simulink model "eVTOL_System"  (R2024b)
settings: Solver=FixedStepAuto  StartTime=0.0  StopTime=inf  RelTol=1e-3
undefined symbols (not defined in the file): airspeed, Battery, BCE12, BCE_Set_init, BMS_Controller_State, C, Cell10_P, Cell11_P, Cell12_P, Cell13_P, Cell14_P, Cell15_P, Cell16_P, Cell17_P, Cell18_P, Cell19_P, Cell1_N, Cell1_P, Cell20_P, Cell21_P, Cell22_P, Cell23_P, Cell24_P, Cell2_P, Cell3_P, Cell4_P, Cell5_P, Cell6_P, Cell7_P, Cell8_P, Cell9_P, Charging_State, CityMission, control, controlParams, ControlSampleTime, CriticalTiltAngle, currentFactor, CV_Gain, ddx, ddy, ddz, Device_01, Device_02, DiscIntNeverNeededParam, dx, dy, dz, Earth, env, F, F28379D_ADC_MaxCount, F28379D_ADC_Vmax, FixedWingMission, flightState, Foc_Ki_IxTcpu, Foc_Ki_S, Foc_Kp_I, Foc_Kp_S, fractalcoef ... (+68)
libraries: fl_lib x1115, nesl_utility x617, slrealtimeethercatlib x217, simulink x130, canmsglib x101, speedgoatlib_IO611_obsolete x91, slpidlib x49, mcbcontrolslib x44, slrealtimeutilitieslib x35, speedgoatlib_hdlCoder_IO3xx x31, dspstat3 x24, mcbpositiondecoderlib x12
(part 19 of 31)

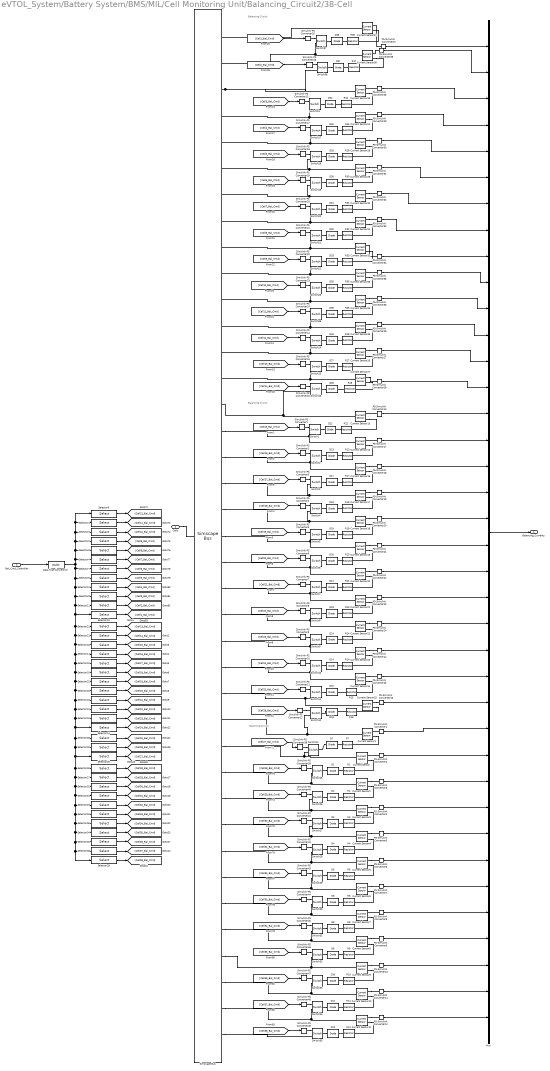
== system eVTOL_System/Battery System/BMS/MIL/Cell Monitoring Unit/Balancing_Circuit2/38-Cell ==
  note: Balancing Circuit
  note: Balancing Circuit
  note: Balancing Circuit
  Bal_Cmd_Controller : Inport
  Current Sensor{,1..37} (38 alike) : fl_lib/Electrical/Electrical Sensors/Current Sensor
  D{1..38} (38 alike) : fl_lib/Electrical/Electrical Elements/Diode  Vf=0.6 V  Ron=0.3 Ohm  Goff=1e-8 1/Ohm  i_specify=off  i_priority=High  i=0 A  i_nominal_specify=off  i_nominal_value=1  i_nominal_unit=A  v_specify=off  v_priority=None  v=0 V  v_nominal_specify=off  v_nominal_value=1  v_nominal_unit=V
      settings: LibrarySourceBlock=BatteryPack_lib/CellMonitoringUnit/D1  LogSimulationData=on
  Data Type Conversion : DataTypeConversion  OutDataTypeStr=double  SaturateOnIntegerOverflow=off  RndMeth=Floor
  Mux : Mux  Inputs=38
  PS-Simulink Converter{1..38} (38 alike) : nesl_utility/PS-Simulink Converter  PhysicalDomain=network_engine_domain  SubClassName=ps_output  LeftPortType=input  RightPortType=output  PseudoPeriodic=off  Frequencies=[]  VectorFormat=inherit  Unit=inherit  AffineConversion=off
  R{1..38} (38 alike) : fl_lib/Electrical/Electrical Elements/Resistor  R=Battery.R_bleed Ohm  i_specify=off  i_priority=None  i=0 A  i_nominal_specify=off  i_nominal_value=1  i_nominal_unit=A  v_specify=off  v_priority=None  v=0 V  v_nominal_specify=off  v_nominal_value=1  v_nominal_unit=V
      settings: LibrarySourceBlock=BatteryPack_lib/CellMonitoringUnit/R1  LogSimulationData=on
  Selector1 : Selector  IndexOptions=Index vector (dialog)  Indices=73  OutputSizes=1
  Selector10 : Selector  IndexOptions=Index vector (dialog)  Indices=63  OutputSizes=1
  Selector11 : Selector  IndexOptions=Index vector (dialog)  Indices=64  OutputSizes=1
  Selector12 : Selector  IndexOptions=Index vector (dialog)  Indices=66  OutputSizes=1
  Selector13 : Selector  IndexOptions=Index vector (dialog)  Indices=76  OutputSizes=1
  Selector14 : Selector  IndexOptions=Index vector (dialog)  Indices=86  OutputSizes=1
  Selector15 : Selector  IndexOptions=Index vector (dialog)  Indices=85  OutputSizes=1
  Selector16 : Selector  IndexOptions=Index vector (dialog)  Indices=83  OutputSizes=1
  Selector17 : Selector  IndexOptions=Index vector (dialog)  Indices=78  OutputSizes=1
  Selector18 : Selector  IndexOptions=Index vector (dialog)  Indices=77  OutputSizes=1
  Selector19 : Selector  IndexOptions=Index vector (dialog)  Indices=80  OutputSizes=1
  Selector2 : Selector  IndexOptions=Index vector (dialog)  Indices=71  OutputSizes=1
  Selector20 : Selector  IndexOptions=Index vector (dialog)  Indices=82  OutputSizes=1
  Selector21 : Selector  IndexOptions=Index vector (dialog)  Indices=75  OutputSizes=1
  Selector22 : Selector  IndexOptions=Index vector (dialog)  Indices=81  OutputSizes=1
  Selector23 : Selector  IndexOptions=Index vector (dialog)  Indices=79  OutputSizes=1
  Selector24 : Selector  IndexOptions=Index vector (dialog)  Indices=84  OutputSizes=1
  Selector25 : Selector  IndexOptions=Index vector (dialog)  Indices=89  OutputSizes=1
  Selector26 : Selector  IndexOptions=Index vector (dialog)  Indices=88  OutputSizes=1
  Selector27 : Selector  IndexOptions=Index vector (dialog)  Indices=91  OutputSizes=1
  Selector29 : Selector  IndexOptions=Index vector (dialog)  Indices=100  OutputSizes=1
  Selector3 : Selector  IndexOptions=Index vector (dialog)  Indices=72  OutputSizes=1
  Selector30 : Selector  IndexOptions=Index vector (dialog)  Indices=98  OutputSizes=1
  Selector31 : Selector  IndexOptions=Index vector (dialog)  Indices=93  OutputSizes=1
  Selector32 : Selector  IndexOptions=Index vector (dialog)  Indices=92  OutputSizes=1
  Selector33 : Selector  IndexOptions=Index vector (dialog)  Indices=95  OutputSizes=1
  Selector34 : Selector  IndexOptions=Index vector (dialog)  Indices=97  OutputSizes=1
  Selector35 : Selector  IndexOptions=Index vector (dialog)  Indices=90  OutputSizes=1
  Selector36 : Selector  IndexOptions=Index vector (dialog)  Indices=96  OutputSizes=1
  Selector37 : Selector  IndexOptions=Index vector (dialog)  Indices=94  OutputSizes=1
  Selector38 : Selector  IndexOptions=Index vector (dialog)  Indices=99  OutputSizes=1
  Selector39 : Selector  IndexOptions=Index vector (dialog)  Indices=87  OutputSizes=1
  Selector4 : Selector  IndexOptions=Index vector (dialog)  Indices=69  OutputSizes=1
  Selector5 : Selector  IndexOptions=Index vector (dialog)  Indices=67  OutputSizes=1
  Selector6 : Selector  IndexOptions=Index vector (dialog)  Indices=74  OutputSizes=1
  Selector7 : Selector  IndexOptions=Index vector (dialog)  Indices=68  OutputSizes=1
  Selector8 : Selector  IndexOptions=Index vector (dialog)  Indices=70  OutputSizes=1
  Selector9 : Selector  IndexOptions=Index vector (dialog)  Indices=65  OutputSizes=1
  Simscape Bus : SimscapeBus  HierarchyStrings=Cell38_P;Cell37_P;Cell36_P;Cell35_P;Cell34_P;Cell33_P;Cell32_P;Cell31_P;Cell30_P;Cell29_P;Cell28_P;Cell27_P;Cell26_P;Cell25_P;Cell24_P;Cell23_P;Cell22_P;Cell21_P;Cell20_P;Cell19_P;Cell18_P;Cell17_P;Cell16_P;Cell15_P;Cell14_P;Cell13_P;Cell12_P;Cell11_P;Cell10_P;Cell9_P;Cell8_P;Cell7_P;Cell6_P;Cell5_P;Cell4_P;Cell3_P;Cell2_P;Cell1_P;Cell1_N
  Simulink-PS Converter{1..26,38..49} (38 alike) : nesl_utility/Simulink-PS Converter  PhysicalDomain=network_engine_domain  SubClassName=ps_input  LeftPortType=input  RightPortType=output  PseudoPeriodic=off  Frequencies=[]  NoiseDistribution=none  NoiseParameters=[]  Unit=1  AffineConversion=off  FilteringAndDerivatives=zero  SimscapeFilterOrder=1  InputFilterTimeConstant=0.001  UdotUserProvided=1
      settings: LibrarySourceBlock=|
      | BatteryPack_lib/CellMonitoringUnit/Simulink-PS
      | Converter3
  Switch{1..38} (38 alike) : fl_lib/Electrical/Electrical Elements/Switch  R_closed=0.01 Ohm  G_open=1e-8 1/Ohm  Threshold=0  i_specify=off  i_priority=None  i=0 A  i_nominal_specify=off  i_nominal_value=1  i_nominal_unit=A  v_specify=off  v_priority=None  v=0 V  v_nominal_specify=off  v_nominal_value=1  v_nominal_unit=V
      settings: LibrarySourceBlock=BatteryPack_lib/CellMonitoringUnit/Switch
  Cells : PMIOPort  Side=Left
  Balancing_Currents : Outport
  wires:
  [Cell36_Bal_Cmd] -> Simulink-PS Converter47/1
  [Cell35_Bal_Cmd] -> Simulink-PS Converter46/1
  [Cell37_Bal_Cmd] -> Simulink-PS Converter48/1
  [Cell30_Bal_Cmd] -> Simulink-PS Converter41/1
  [Cell33_Bal_Cmd] -> Simulink-PS Converter44/1
  [Cell28_Bal_Cmd] -> Simulink-PS Converter39/1
  [Cell38_Bal_Cmd] -> Simulink-PS Converter49/1
  [Cell29_Bal_Cmd] -> Simulink-PS Converter40/1
  [Cell31_Bal_Cmd] -> Simulink-PS Converter42/1
  [Cell32_Bal_Cmd] -> Simulink-PS Converter43/1
  [Cell34_Bal_Cmd] -> Simulink-PS Converter45/1
  Selector11/1 -> [Cell2_Bal_Cmd]
  Selector12/1 -> [Cell4_Bal_Cmd]
  Selector3/1 -> [Cell10_Bal_Cmd]
  Selector9/1 -> [Cell3_Bal_Cmd]
  Selector1/1 -> [Cell11_Bal_Cmd]
  Selector4/1 -> [Cell7_Bal_Cmd]
  Selector8/1 -> [Cell8_Bal_Cmd]
  Selector6/1 -> [Cell12_Bal_Cmd]
  Selector7/1 -> [Cell6_Bal_Cmd]
  Selector5/1 -> [Cell5_Bal_Cmd]
  Selector10/1 -> [Cell1_Bal_Cmd]
  Selector2/1 -> [Cell9_Bal_Cmd]
  Bal_Cmd_Controller/1 -> Data Type Conversion/1
  Mux/1 -> Balancing_Currents/1
  [Cell19_Bal_Cmd] -> Simulink-PS Converter5/1
  [Cell20_Bal_Cmd] -> Simulink-PS Converter6/1
  [Cell16_Bal_Cmd] -> Simulink-PS Converter2/1
  [Cel15_Bal_Cmd] -> Simulink-PS Converter1/1
  [Cell21_Bal_Cmd] -> Simulink-PS Converter7/1
  [Cell22_Bal_Cmd] -> Simulink-PS Converter8/1
  [Cell17_Bal_Cmd] -> Simulink-PS Converter3/1
  [Cell23_Bal_Cmd] -> Simulink-PS Converter9/1
  [Cell18_Bal_Cmd] -> Simulink-PS Converter4/1
  [Cell24_Bal_Cmd] -> Simulink-PS Converter10/1
  Selector13/1 -> [Cell14_Bal_Cmd]
  Selector20/1 -> [Cell20_Bal_Cmd]
  Selector22/1 -> [Cell19_Bal_Cmd]
  Selector15/1 -> [Cell23_Bal_Cmd]
  Selector17/1 -> [Cell16_Bal_Cmd]
  Selector23/1 -> [Cell17_Bal_Cmd]
  Selector18/1 -> [Cell15_Bal_Cmd]
  Selector16/1 -> [Cell21_Bal_Cmd]
  Selector14/1 -> [Cell24_Bal_Cmd]
  Selector21/1 -> [Cell13_Bal_Cmd]
  Selector24/1 -> [Cell22_Bal_Cmd]
  Selector19/1 -> [Cell18_Bal_Cmd]
  Selector35/1 -> [Cell28_Bal_Cmd]
  Selector30/1 -> [Cell36_Bal_Cmd]
  Selector29/1 -> [Cell38_Bal_Cmd]
  Selector38/1 -> [Cell37_Bal_Cmd]
  Selector32/1 -> [Cell30_Bal_Cmd]
  Selector33/1 -> [Cell33_Bal_Cmd]
  Selector34/1 -> [Cell35_Bal_Cmd]
  Selector37/1 -> [Cell32_Bal_Cmd]
  Selector39/1 -> [Cell25_Bal_Cmd]
  Selector25/1 -> [Cell27_Bal_Cmd]
  Data Type Conversion/1 -> Selector4/1, Selector8/1, Selector2/1, Selector3/1, Selector1/1, Selector6/1, Selector7/1, Selector5/1, Selector12/1, Selector9/1, Selector11/1, Selector30/1, Selector29/1, Selector38/1, Selector34/1, Selector36/1, Selector33/1, Selector37/1, Selector31/1, Selector32/1, Selector27/1, Selector35/1, Selector25/1, Selector26/1, Selector39/1, Selector14/1, Selector15/1, Selector24/1, Selector16/1, Selector20/1, Selector22/1, Selector19/1, Selector23/1, Selector17/1, Selector18/1, Selector13/1, Selector21/1, Selector10/1
  Selector36/1 -> [Cell34_Bal_Cmd]
  Selector27/1 -> [Cell29_Bal_Cmd]
  Selector31/1 -> [Cell31_Bal_Cmd]
  Selector26/1 -> [Cell26_Bal_Cmd]
  [Cell6_Bal_Cmd] -> Simulink-PS Converter19/1
  [Cell10_Bal_Cmd] -> Simulink-PS Converter23/1
  [Cell11_Bal_Cmd] -> Simulink-PS Converter24/1
  [Cell8_Bal_Cmd] -> Simulink-PS Converter21/1
  [Cell13_Bal_Cmd] -> Simulink-PS Converter15/1
  [Cell12_Bal_Cmd] -> Simulink-PS Converter14/1
  [Cell9_Bal_Cmd] -> Simulink-PS Converter22/1
  [Cell3_Bal_Cmd] -> Simulink-PS Converter13/1
  [Cell5_Bal_Cmd] -> Simulink-PS Converter18/1
  [Cell4_Bal_Cmd] -> Simulink-PS Converter17/1
  [Cell7_Bal_Cmd] -> Simulink-PS Converter20/1
  [Cell1_Bal_Cmd] -> Simulink-PS Converter25/1
  [Cell2_Bal_Cmd] -> Simulink-PS Converter26/1
  PS-Simulink Converter37/1 -> Mux/1
  PS-Simulink Converter38/1 -> Mux/2
  PS-Simulink Converter34/1 -> Mux/9
  PS-Simulink Converter33/1 -> Mux/8
  PS-Simulink Converter35/1 -> Mux/10
  PS-Simulink Converter32/1 -> Mux/7
  PS-Simulink Converter36/1 -> Mux/11
  PS-Simulink Converter31/1 -> Mux/6
  PS-Simulink Converter26/1 -> Mux/12
  PS-Simulink Converter30/1 -> Mux/5
  PS-Simulink Converter27/1 -> Mux/13
  PS-Simulink Converter29/1 -> Mux/4
  PS-Simulink Converter28/1 -> Mux/14
  PS-Simulink Converter25/1 -> Mux/3
  PS-Simulink Converter18/1 -> Mux/17
  PS-Simulink Converter17/1 -> Mux/16
  PS-Simulink Converter19/1 -> Mux/18
  PS-Simulink Converter13/1 -> Mux/15
  PS-Simulink Converter20/1 -> Mux/19
  PS-Simulink Converter21/1 -> Mux/20
  PS-Simulink Converter22/1 -> Mux/21
  PS-Simulink Converter23/1 -> Mux/22
  PS-Simulink Converter24/1 -> Mux/23
  PS-Simulink Converter14/1 -> Mux/24
  PS-Simulink Converter15/1 -> Mux/25
  PS-Simulink Converter16/1 -> Mux/26
  PS-Simulink Converter1/1 -> Mux/27
  PS-Simulink Converter2/1 -> Mux/28
  PS-Simulink Converter3/1 -> Mux/29
  PS-Simulink Converter4/1 -> Mux/30
  PS-Simulink Converter5/1 -> Mux/31
  PS-Simulink Converter6/1 -> Mux/32
  PS-Simulink Converter7/1 -> Mux/33
  PS-Simulink Converter8/1 -> Mux/34
  PS-Simulink Converter9/1 -> Mux/35
  PS-Simulink Converter10/1 -> Mux/36
  PS-Simulink Converter11/1 -> Mux/37
  PS-Simulink Converter12/1 -> Mux/38
  [Cell14_Bal_Cmd] -> Simulink-PS Converter16/1
  [Cell25_Bal_Cmd] -> Simulink-PS Converter11/1
  [Cell26_Bal_Cmd] -> Simulink-PS Converter12/1
  [Cell27_Bal_Cmd] -> Simulink-PS Converter38/1
  connections:
  Current Sensor5/LConn1 -- Simscape Bus/LConn32 -- Switch28/RConn2
  Current Sensor2/LConn1 -- Simscape Bus/LConn29 -- Switch25/RConn2
  Simscape Bus/LConn31 -- Current Sensor4/LConn1 -- Switch27/RConn2
  Current Sensor11/LConn1 -- Simscape Bus/LConn38 -- Switch34/RConn2
  Simscape Bus/LConn30 -- Current Sensor3/LConn1 -- Switch26/RConn2
  Current Sensor9/LConn1 -- Simscape Bus/LConn36 -- Switch32/RConn2
  Current Sensor7/LConn1 -- Simscape Bus/LConn34 -- Switch30/RConn2
  Current Sensor/LConn1 -- Simscape Bus/LConn28 -- Switch24/RConn2
  Current Sensor8/LConn1 -- Simscape Bus/LConn35 -- Switch31/RConn2
  Current Sensor6/LConn1 -- Simscape Bus/LConn33 -- Switch29/RConn2
  Current Sensor10/LConn1 -- Simscape Bus/LConn37 -- Switch33/RConn2
  Simulink-PS Converter38/RConn1 -- Switch24/RConn1
  R4/RConn1 -- D4/LConn1
  Simulink-PS Converter48/RConn1 -- Switch34/RConn1
  R7/RConn1 -- D7/LConn1
  R8/RConn1 -- D8/LConn1
  Switch25/LConn1 -- D1/RConn1
  R6/RConn1 -- D6/LConn1
  R10/RConn1 -- D10/LConn1
  R12/RConn1 -- D12/LConn1
  Simulink-PS Converter49/RConn1 -- Switch35/RConn1
  R11/RConn1 -- D11/LConn1
  Switch30/LConn1 -- D6/RConn1
  Simulink-PS Converter41/RConn1 -- Switch27/RConn1
  Switch32/LConn1 -- D9/RConn1
  Switch31/LConn1 -- D8/RConn1
  Simulink-PS Converter39/RConn1 -- Switch25/RConn1
  Switch24/LConn1 -- D7/RConn1
  Simulink-PS Converter47/RConn1 -- Switch33/RConn1
  Simulink-PS Converter46/RConn1 -- Switch32/RConn1
  Switch35/LConn1 -- D12/RConn1
  Switch29/LConn1 -- D5/RConn1
  R2/RConn1 -- D2/LConn1
  Simulink-PS Converter44/RConn1 -- Switch30/RConn1
  Switch27/LConn1 -- D3/RConn1
  Switch28/LConn1 -- D4/RConn1
  Simulink-PS Converter43/RConn1 -- Switch29/RConn1
  Simulink-PS Converter45/RConn1 -- Switch31/RConn1
  R3/RConn1 -- D3/LConn1
  R9/RConn1 -- D9/LConn1
  Simulink-PS Converter42/RConn1 -- Switch28/RConn1
  Switch26/LConn1 -- D2/RConn1
  Simulink-PS Converter40/RConn1 -- Switch26/RConn1
  R5/RConn1 -- D5/LConn1
  Switch33/LConn1 -- D10/RConn1
  Switch34/LConn1 -- D11/RConn1
  R1/RConn1 -- D1/LConn1
  Simscape Bus/LConn39 -- Switch35/RConn2
  Current Sensor1/LConn1 -- Simscape Bus/LConn27 -- Switch12/RConn2
  Current Sensor1/RConn2 -- R7/LConn1
  Current Sensor2/RConn2 -- R2/LConn1
  Current Sensor3/RConn2 -- R3/LConn1
  Current Sensor4/RConn2 -- R4/LConn1
  Current Sensor5/RConn2 -- R5/LConn1
  Current Sensor6/RConn2 -- R6/LConn1
  Current Sensor7/RConn2 -- R8/LConn1
  Current Sensor8/RConn2 -- R9/LConn1
  Current Sensor9/RConn2 -- R10/LConn1
  Current Sensor10/RConn2 -- R11/LConn1
  Current Sensor11/RConn2 -- R12/LConn1
  Current Sensor/RConn2 -- R1/LConn1
  PS-Simulink Converter1/LConn1 -- Current Sensor1/RConn1
  PS-Simulink Converter2/LConn1 -- Current Sensor/RConn1
  Current Sensor2/RConn1 -- PS-Simulink Converter3/LConn1
  Current Sensor3/RConn1 -- PS-Simulink Converter4/LConn1
  PS-Simulink Converter8/LConn1 -- Current Sensor7/RConn1
  Current Sensor6/RConn1 -- PS-Simulink Converter7/LConn1
  Current Sensor5/RConn1 -- PS-Simulink Converter6/LConn1
  Current Sensor4/RConn1 -- PS-Simulink Converter5/LConn1
  Current Sensor8/RConn1 -- PS-Simulink Converter9/LConn1
  Current Sensor9/RConn1 -- PS-Simulink Converter10/LConn1
  Current Sensor10/RConn1 -- PS-Simulink Converter11/LConn1
  Current Sensor11/RConn1 -- PS-Simulink Converter12/LConn1
  Current Sensor21/LConn1 -- Switch7/RConn2 -- Simscape Bus/LConn22
  Current Sensor16/LConn1 -- Switch2/RConn2 -- Simscape Bus/LConn17
  Current Sensor17/LConn1 -- Switch3/RConn2 -- Simscape Bus/LConn18
  Current Sensor22/LConn1 -- Switch8/RConn2 -- Simscape Bus/LConn23
  Current Sensor20/LConn1 -- Switch6/RConn2 -- Simscape Bus/LConn21
  Current Sensor23/LConn1 -- Switch9/RConn2 -- Simscape Bus/LConn24
  Current Sensor14/LConn1 -- Switch10/RConn2 -- Simscape Bus/LConn25
  Current Sensor12/LConn1 -- Switch1/RConn2 -- Simscape Bus/LConn16
  Current Sensor19/LConn1 -- Switch5/RConn2 -- Simscape Bus/LConn20
  Current Sensor15/LConn1 -- Switch11/RConn2 -- Simscape Bus/LConn26
  Current Sensor18/LConn1 -- Switch4/RConn2 -- Simscape Bus/LConn19
  Current Sensor20/RConn1 -- PS-Simulink Converter22/LConn1
  Switch8/LConn1 -- D23/RConn1
  Simulink-PS Converter6/RConn1 -- Switch6/RConn1
  PS-Simulink Converter13/LConn1 -- Current Sensor13/RConn1
  Current Sensor15/RConn1 -- PS-Simulink Converter16/LConn1
  Simulink-PS Converter9/RConn1 -- Switch9/RConn1
  R17/RConn1 -- D17/LConn1
  Current Sensor18/RConn2 -- R19/LConn1
  Current Sensor12/RConn2 -- R13/LConn1
  Current Sensor19/RConn2 -- R20/LConn1
  PS-Simulink Converter17/LConn1 -- Current Sensor12/RConn1
  Simulink-PS Converter5/RConn1 -- Switch5/RConn1
  Current Sensor22/RConn2 -- R24/LConn1
  Switch7/LConn1 -- D21/RConn1
  Current Sensor13/RConn2 -- R22/LConn1
  Switch4/LConn1 -- D18/RConn1
  Current Sensor23/RConn2 -- R14/LConn1
  Current Sensor21/RConn2 -- R23/LConn1
  R19/RConn1 -- D19/LConn1
  Current Sensor14/RConn2 -- R15/LConn1
  Current Sensor22/RConn1 -- PS-Simulink Converter24/LConn1
  Simulink-PS Converter1/RConn1 -- Switch1/RConn1
  Simulink-PS Converter2/RConn1 -- Switch2/RConn1
  Switch3/LConn1 -- D17/RConn1
  Simulink-PS Converter8/RConn1 -- Switch8/RConn1
  Current Sensor23/RConn1 -- PS-Simulink Converter14/LConn1
  Switch12/LConn1 -- D16/RConn1
  Switch2/LConn1 -- D13/RConn1
  Current Sensor16/RConn2 -- R17/LConn1
  Current Sensor18/RConn1 -- PS-Simulink Converter20/LConn1
  R14/RConn1 -- D14/LConn1
  Simulink-PS Converter11/RConn1 -- Switch11/RConn1
  R20/RConn1 -- D20/LConn1
  Switch16/RConn2 -- Current Sensor13/LConn1 -- Simscape Bus/LConn15
  Current Sensor19/RConn1 -- PS-Simulink Converter21/LConn1
  R15/RConn1 -- D15/LConn1
  Simulink-PS Converter7/RConn1 -- Switch7/RConn1
  Simulink-PS Converter10/RConn1 -- Switch10/RConn1
  Current Sensor15/RConn2 -- R16/LConn1
  Switch11/LConn1 -- D15/RConn1
  Simulink-PS Converter4/RConn1 -- Switch4/RConn1
  Switch10/LConn1 -- D14/RConn1
  Current Sensor14/RConn1 -- PS-Simulink Converter15/LConn1
  Switch5/LConn1 -- D19/RConn1
  R24/RConn1 -- D24/LConn1
  R21/RConn1 -- D21/LConn1
  Current Sensor16/RConn1 -- PS-Simulink Converter18/LConn1
  R22/RConn1 -- D22/LConn1
  R18/RConn1 -- D18/LConn1
  Switch9/LConn1 -- D24/RConn1
  Switch6/LConn1 -- D20/RConn1
  PS-Simulink Converter23/LConn1 -- Current Sensor21/RConn1
  Switch1/LConn1 -- D22/RConn1
  Current Sensor20/RConn2 -- R21/LConn1
  Simulink-PS Converter3/RConn1 -- Switch3/RConn1
  R23/RConn1 -- D23/LConn1
  Simulink-PS Converter12/RConn1 -- Switch12/RConn1
  R16/RConn1 -- D16/LConn1
  R13/RConn1 -- D13/LConn1
  Current Sensor17/RConn1 -- PS-Simulink Converter19/LConn1
  Current Sensor17/RConn2 -- R18/LConn1
  Cells/RConn1 -- Simscape Bus/RConn1
  Current Sensor31/LConn1 -- Switch20/RConn2 -- Simscape Bus/LConn8
  Current Sensor26/LConn1 -- Switch14/RConn2 -- Simscape Bus/LConn13
  Current Sensor30/LConn1 -- Switch19/RConn2 -- Simscape Bus/LConn7
  Current Sensor35/LConn1 -- Switch36/RConn2 -- Simscape Bus/LConn12
  Current Sensor32/LConn1 -- Switch21/RConn2 -- Simscape Bus/LConn9
  Current Sensor27/LConn1 -- Switch15/RConn2 -- Simscape Bus/LConn14
  Current Sensor33/LConn1 -- Switch22/RConn2 -- Simscape Bus/LConn10
  Current Sensor29/LConn1 -- Switch18/RConn2 -- Simscape Bus/LConn6
  Current Sensor34/LConn1 -- Switch23/RConn2 -- Simscape Bus/LConn11
  Current Sensor28/LConn1 -- Switch17/RConn2 -- Simscape Bus/LConn5
  Current Sensor24/LConn1 -- Switch13/RConn2 -- Simscape Bus/LConn4
  Switch13/LConn1 -- D34/RConn1
  Switch36/LConn1 -- D36/RConn1
  Simulink-PS Converter23/RConn1 -- Switch23/RConn1
  Switch16/LConn1 -- D28/RConn1
  Current Sensor27/RConn1 -- PS-Simulink Converter28/LConn1
  Current Sensor29/RConn2 -- R30/LConn1
  Current Sensor34/RConn1 -- PS-Simulink Converter36/LConn1
  Simulink-PS Converter20/RConn1 -- Switch20/RConn1
  R31/RConn1 -- D31/LConn1
  R25/RConn1 -- D25/LConn1
  Current Sensor31/RConn2 -- R32/LConn1
  Simulink-PS Converter18/RConn1 -- Switch18/RConn1
  Current Sensor26/RConn2 -- R27/LConn1
  Current Sensor31/RConn1 -- PS-Simulink Converter33/LConn1
  R30/RConn1 -- D30/LConn1
  Current Sensor26/RConn1 -- PS-Simulink Converter27/LConn1
  Current Sensor30/RConn2 -- R31/LConn1
  Current Sensor27/RConn2 -- R28/LConn1
  Current Sensor32/RConn2 -- R33/LConn1
  Switch20/LConn1 -- D31/RConn1
  Simulink-PS Converter22/RConn1 -- Switch22/RConn1
  Simulink-PS Converter15/RConn1 -- Switch15/RConn1
  PS-Simulink Converter29/LConn1 -- Current Sensor24/RConn1
  R32/RConn1 -- D32/LConn1
  Simulink-PS Converter17/RConn1 -- Switch17/RConn1
  Current Sensor30/RConn1 -- PS-Simulink Converter32/LConn1
  Switch14/LConn1 -- D26/RConn1
  Switch17/LConn1 -- D25/RConn1
  R35/RConn1 -- D35/LConn1
  R27/RConn1 -- D27/LConn1
  Simulink-PS Converter21/RConn1 -- Switch21/RConn1
  Switch22/LConn1 -- D33/RConn1
  Simulink-PS Converter14/RConn1 -- Switch14/RConn1
  Simulink-PS Converter19/RConn1 -- Switch19/RConn1
  R36/RConn1 -- D36/LConn1
  Current Sensor34/RConn2 -- R36/LConn1
  PS-Simulink Converter35/LConn1 -- Current Sensor33/RConn1
  Simscape Bus/LConn3 -- Current Sensor25/LConn1 -- Switch38/RConn2
  Switch23/LConn1 -- D35/RConn1
  PS-Simulink Converter25/LConn1 -- Current Sensor25/RConn1
  Simulink-PS Converter13/RConn1 -- Switch13/RConn1
  R26/RConn1 -- D26/LConn1
  R28/RConn1 -- D28/LConn1
  Simulink-PS Converter16/RConn1 -- Switch16/RConn1
  Switch18/LConn1 -- D29/RConn1
  Current Sensor35/RConn2 -- R26/LConn1
  R33/RConn1 -- D33/LConn1
  Current Sensor28/RConn1 -- PS-Simulink Converter30/LConn1
  Current Sensor24/RConn2 -- R25/LConn1
  Current Sensor32/RConn1 -- PS-Simulink Converter34/LConn1
  Current Sensor28/RConn2 -- R29/LConn1
  R34/RConn1 -- D34/LConn1
  Switch19/LConn1 -- D30/RConn1
  Simulink-PS Converter24/RConn1 -- Switch36/RConn1
  Switch21/LConn1 -- D32/RConn1
  Switch15/LConn1 -- D27/RConn1
  Current Sensor33/RConn2 -- R35/LConn1
  R29/RConn1 -- D29/LConn1
  Current Sensor29/RConn1 -- PS-Simulink Converter31/LConn1
  Current Sensor35/RConn1 -- PS-Simulink Converter26/LConn1
  Current Sensor25/RConn2 -- R34/LConn1
  Current Sensor36/LConn1 -- Switch37/RConn2 -- Simscape Bus/LConn2
  Switch38/LConn1 -- D37/RConn1
  R38/RConn1 -- D38/LConn1
  PS-Simulink Converter37/LConn1 -- Current Sensor37/RConn1
  R37/RConn1 -- D37/LConn1
  Current Sensor36/RConn2 -- R37/LConn1
  Switch37/LConn1 -- D38/RConn1
  Current Sensor37/LConn1 -- Simscape Bus/LConn1
  Simulink-PS Converter26/RConn1 -- Switch38/RConn1
  PS-Simulink Converter38/LConn1 -- Current Sensor36/RConn1
  Simulink-PS Converter25/RConn1 -- Switch37/RConn1
  Current Sensor37/RConn2 -- R38/LConn1

== system eVTOL_System/Battery System/BMS/MIL/Controller/Current Calculations/Charge_Current_Limit_Calc ==
  MaxCellVolt : Inport
  MinCellTemp : Inport  Port=2
  MaxCellTemp : Inport  Port=3
  Divide1 : Product  Inputs=*/
  HighTempChrgCurrentLim : Lookup_n-D  NumberOfTableDimensions=1  BreakpointsForDimension1=273.15+[-30:1:70]  Table=50*(1-tanh(273.15+[-30:1:70]-273.15-50))/2  InternalRulePriority=Speed  RndMeth=Simplest
  InternalCellResistance : Constant  Value=single(max(max(Battery(1).R0_LUT)))  OutDataTypeStr=single  SampleTime=-1
  LowTempChrgCurrentLim : Lookup_n-D  NumberOfTableDimensions=1  BreakpointsForDimension1=273.15+[-30:1:70]  Table=50*(1+tanh(273.15+[-30:1:70]-(273.15)))/2  InternalRulePriority=Speed  RndMeth=Simplest
  MinMax2 : MinMax  Inputs=3
  OverVoltageLimit : Constant  Value=OverCellVoltageLimit  OutDataTypeStr=single  SampleTime=-1
  Subtract1 : Sum  Inputs=+-
  Charge_Current_Limit : Outport  VectorParamsAs1DForOutWhenUnconnected=off
  wires:
  OverVoltageLimit/1 -> Subtract1/1
  MinMax2/1 -> Charge_Current_Limit/1  "ChargeCurrentLimit"
  MaxCellVolt/1 -> Subtract1/2
  Subtract1/1 -> Divide1/1
  Divide1/1 -> MinMax2/1
  InternalCellResistance/1 -> Divide1/2
  MinCellTemp/1 -> LowTempChrgCurrentLim/1
  MaxCellTemp/1 -> HighTempChrgCurrentLim/1
  HighTempChrgCurrentLim/1 -> MinMax2/3
  LowTempChrgCurrentLim/1 -> MinMax2/2

== system eVTOL_System/Battery System/BMS/MIL/Controller/Current Calculations/Discharge_Current_Limit_Calc ==
  MinCellVolt : Inport
  MinCellTemp : Inport  Port=2
  MaxCellTemp : Inport  Port=3
  Divide : Product  Inputs=*/
  Gain : Gain  Gain=-1
  HighTempDchrgCurrentLim : Lookup_n-D  NumberOfTableDimensions=1  BreakpointsForDimension1=273.15+[-30:1:70]  Table=100*(1-tanh(273.15+[-30:1:70]-273.15-50))/2  InternalRulePriority=Speed  RndMeth=Simplest
  InternalCellResistance : Constant  Value=single(max(max(Battery(1).R0_LUT)))  OutDataTypeStr=single  SampleTime=-1
  LowTempDchrgCurrentLim : Lookup_n-D  NumberOfTableDimensions=1  BreakpointsForDimension1=273.15+[-30:1:70]  Table=100*(1+tanh(273.15+[-30:1:70]-(273.15)))/2  InternalRulePriority=Speed  RndMeth=Simplest
  MinMax2 : MinMax  Inputs=3
  Subtract : Sum  Inputs=+-
  UnderVoltageLimit : Constant  Value=UnderCellVoltageLimit  OutDataTypeStr=single  SampleTime=-1
  Discharge_Current_Limit : Outport  VectorParamsAs1DForOutWhenUnconnected=off
  wires:
  MinMax2/1 -> Gain/1  "DischargeCurrentLimit"
  Divide/1 -> MinMax2/1
  MinCellVolt/1 -> Subtract/1
  InternalCellResistance/1 -> Divide/2
  Subtract/1 -> Divide/1
  UnderVoltageLimit/1 -> Subtract/2
  Gain/1 -> Discharge_Current_Limit/1
  MaxCellTemp/1 -> HighTempDchrgCurrentLim/1
  MinCellTemp/1 -> LowTempDchrgCurrentLim/1
  HighTempDchrgCurrentLim/1 -> MinMax2/3
  LowTempDchrgCurrentLim/1 -> MinMax2/2

== system eVTOL_System/Battery System/BMS/MIL/Controller/SOC Calculation/Coulomb Counting ==
  Curr : Inport
  Temp : Inport  Port=2
  1-D Lookup Table : Lookup_n-D  NumberOfTableDimensions=1  BreakpointsForDimension1=single(Battery(1).Temperature_LUT)  Table=single(Battery(1).Capacity_LUT)  InternalRulePriority=Speed  RndMeth=Simplest
  Discrete-Time Integrator : DiscreteIntegrator  InitialCondition=single(SOCInit+0.05)  SampleTime=-1  LimitOutput=on  UpperSaturationLimit=1  LowerSaturationLimit=0  ICPrevOutput=DiscIntNeverNeededParam  ICPrevScaledInput=DiscIntNeverNeededParam
  Divide : Product  Inputs=*/
  Gain : Gain  Gain=single(1/3600)
  SOC : Outport  VectorParamsAs1DForOutWhenUnconnected=off
  wires:
  Discrete-Time Integrator/1 -> SOC/1
  Curr/1 -> Gain/1
  Gain/1 -> Divide/1
  Divide/1 -> Discrete-Time Integrator/1
  1-D Lookup Table/1 -> Divide/2  "Capacity"
  Temp/1 -> 1-D Lookup Table/1

== system eVTOL_System/Battery System/BMS/MIL/Controller/SOC Calculation/Measurement Function ==
  Current : Inport
  Temperature (K) : Inport  Port=2
  batteryMeasurementFcn : TriggerPort  TriggerType=function-call  IsSimulinkFunction=on  FunctionName=batteryMeasurementFcn  VariantControl=Variant
  Add1 : Sum  Inputs=+--
  Em Table : Lookup_n-D  BreakpointsForDimension1=Battery.SOC_LUT  BreakpointsForDimension2=Battery.Temperature_LUT  BeginIndexSearchUsingPreviousIndexResult=on  Table=Battery.Em_LUT  ExtrapMethod=Clip  InternalRulePriority=Speed  RndMeth=Simplest
      settings: InputPortMap=u0,u1
  Get SOC : Selector  InputPortWidth=2  IndexOptions=Index vector (dialog)  Indices=[1]  OutputSizes=1
  Get U1 : Selector  InputPortWidth=2  IndexOptions=Index vector (dialog)  Indices=2  OutputSizes=1
  Product : Product
  R0 Table : Lookup_n-D  BreakpointsForDimension1=Battery.SOC_LUT  BreakpointsForDimension2=Battery.Temperature_LUT  BeginIndexSearchUsingPreviousIndexResult=on  Table=Battery.R0_LUT  ExtrapMethod=Clip  InternalRulePriority=Speed  RndMeth=Simplest
      settings: InputPortMap=u0,u1
  x : ArgIn  DisableCoverage=on  OutDataTypeStr=single  PortDimensions=2  ArgumentName=x
  y : ArgOut  DisableCoverage=on  OutDataTypeStr=single  ArgumentName=y
  wires:
  Get U1/1 -> Add1/3  "U1"
  Product/1 -> Add1/2
  Current/1 -> Product/2
  R0 Table/1 -> Product/1
  Temperature (K)/1 -> Em Table/2, R0 Table/2
  Add1/1 -> y/1
  Em Table/1 -> Add1/1
  Get SOC/1 -> Em Table/1, R0 Table/1  "SOC"
  x/1 -> Get SOC/1, Get U1/1

== system eVTOL_System/Battery System/BMS/MIL/Controller/SOC Calculation/State Transition Function ==
  Current : Inport
  Temperature K : Inport  Port=2
  batteryStateFcn : TriggerPort  TriggerType=function-call  IsSimulinkFunction=on  FunctionName=batteryStateFcn  VariantControl=Variant
  Add : Sum
  Add1 : Sum  Inputs=-+
  C1 : Lookup_n-D  BreakpointsForDimension1=Battery.SOC_LUT  BreakpointsForDimension2=Battery.Temperature_LUT  BeginIndexSearchUsingPreviousIndexResult=on  Table=Battery.C1_LUT  ExtrapMethod=Clip  InternalRulePriority=Speed  RndMeth=Simplest
      settings: InputPortMap=u0,u1
  Constant : Constant  Value=single(ts_system)  OutDataTypeStr=single
  Divide : Product  Inputs=*/
  Divide1 : Product  Inputs=*/
  Divide2 : Product  Inputs=*/
  Gain : Gain  Gain=-3600
  Get SOC : Selector  InputPortWidth=2  IndexOptions=Index vector (dialog)  Indices=1  OutputSizes=1
  Get U1 : Selector  InputPortWidth=2  IndexOptions=Index vector (dialog)  Indices=2  OutputSizes=1
  Lookup Table : Lookup_n-D  NumberOfTableDimensions=1  BreakpointsForDimension1=Battery.Temperature_LUT  BeginIndexSearchUsingPreviousIndexResult=on  Table=Battery.Capacity_LUT  InternalRulePriority=Speed  RndMeth=Simplest
  Mux : Mux  Inputs=2
  Product : Product  OutDataTypeStr=single
  Product1 : Product
  R1 : Lookup_n-D  BreakpointsForDimension1=Battery.SOC_LUT  BreakpointsForDimension2=Battery.Temperature_LUT  BeginIndexSearchUsingPreviousIndexResult=on  Table=Battery.R1_LUT  ExtrapMethod=Clip  InternalRulePriority=Speed  RndMeth=Simplest
      settings: InputPortMap=u0,u1
  x : ArgIn  DisableCoverage=on  OutDataTypeStr=single  PortDimensions=2  ArgumentName=x
  xNext : ArgOut  DisableCoverage=on  OutDataTypeStr=single  PortDimensions=2  ArgumentName=xNext
  wires:
  Lookup Table/1 -> Gain/1  "Cq"
  Product/1 -> Add/2
  Constant/1 -> Product/2
  Current/1 -> Divide1/1, Divide/1  "Current"
  Get SOC/1 -> C1/1, R1/1
  Temperature K/1 -> Lookup Table/1, C1/2, R1/2
  Add/1 -> xNext/1
  x/1 -> Add/1, Get U1/1, Get SOC/1
  Gain/1 -> Divide/2
  Divide/1 -> Mux/1  "xdot_1"
  Get U1/1 -> Divide2/1  "U1"
  Product1/1 -> Divide2/2  "R1*C1"
  R1/1 -> Product1/1  "R1"
  C1/1 -> Product1/2, Divide1/2  "C1"
  Divide1/1 -> Add1/2  "Current/C1"
  Divide2/1 -> Add1/1
  Add1/1 -> Mux/2  "xdot_2"
  Mux/1 -> Product/1  "xdot"

== system eVTOL_System/Battery System/BMS/MIL/Controller/SOC Calculation/UKF_EKF_1TC ==
  Cell_Voltage : Inport
  Enable : EnablePort
  EKF : sharedTrackingLibrary/Extended Kalman Filter  StateTransitionFcn=batteryStateFcn  HasStateTransitionJacobianFcn=off  HasAdditiveProcessNoise=Additive  ProcessNoise=1e-10*eye(2)  HasTimeVaryingProcessNoise=off  HasStateTransitionFcnExtraArgument=0  InitialState=[single(SOCInit+0.05); 0;]  InitialStateCovariance=[1e-5 1]  MeasurementFcn1=batteryMeasurementFcn  HasMeasurementJacobianFcn1=off  HasMeasurementEnablePort1=off  HasAdditiveMeasurementNoise1=Additive  MeasurementNoise1=1e-1  HasTimeVaryingMeasurementNoise1=off  HasMeasurementFcnExtraArgument1=0  HasMeasurementWrapping1=off  MeasurementFcn2=myMeasurementFcn  HasMeasurementJacobianFcn2=off  HasMeasurementEnablePort2=off  HasAdditiveMeasurementNoise2=Additive  MeasurementNoise2=1  HasTimeVaryingMeasurementNoise2=off  HasMeasurementFcnExtraArgument2=0  HasMeasurementWrapping2=off  MeasurementFcn3=myMeasurementFcn  HasMeasurementJacobianFcn3=off  HasMeasurementEnablePort3=off  HasAdditiveMeasurementNoise3=Additive  MeasurementNoise3=1  HasTimeVaryingMeasurementNoise3=off  HasMeasurementFcnExtraArgument3=0  HasMeasurementWrapping3=off  MeasurementFcn4=myMeasurementFcn  HasMeasurementJacobianFcn4=off  HasMeasurementEnablePort4=off  HasAdditiveMeasurementNoise4=Additive  MeasurementNoise4=1  HasTimeVaryingMeasurementNoise4=off  HasMeasurementFcnExtraArgument4=0  HasMeasurementWrapping4=off  MeasurementFcn5=myMeasurementFcn  HasMeasurementJacobianFcn5=off  HasMeasurementEnablePort5=off  HasAdditiveMeasurementNoise5=Additive  MeasurementNoise5=1  HasTimeVaryingMeasurementNoise5=off  HasMeasurementFcnExtraArgument5=0  HasMeasurementWrapping5=off  EnableMultirate=off  StateTransitionFcnSampleTime=1  MeasurementFcn1SampleTime=1  MeasurementFcn2SampleTime=1  MeasurementFcn3SampleTime=1  MeasurementFcn4SampleTime=1  MeasurementFcn5SampleTime=1  UseCurrentEstimator=on  OutputStateCovariance=off  DataType=single  SampleTime=ts_controller  NumberOfMeasurements=1
  SOC : Selector  InputPortWidth=2  IndexOptions=Index vector (dialog)  Indices=1  OutputSizes=1
  SOC1 : Selector  InputPortWidth=2  IndexOptions=Index vector (dialog)  Indices=1  OutputSizes=1
  UKF : sharedTrackingLibrary/Unscented Kalman Filter  StateTransitionFcn=batteryStateFcn  HasAdditiveProcessNoise=Additive  ProcessNoise=1e-10*eye(2)  HasTimeVaryingProcessNoise=off  HasStateTransitionFcnExtraArgument=0  InitialState=[single(SOCInit+0.05); 0;]  InitialStateCovariance=[1e-5 1]  Alpha=1  Beta=2  Kappa=1  MeasurementFcn1=batteryMeasurementFcn  HasMeasurementEnablePort1=off  HasAdditiveMeasurementNoise1=Additive  MeasurementNoise1=0.1  HasTimeVaryingMeasurementNoise1=off  HasMeasurementFcnExtraArgument1=0  HasMeasurementWrapping1=off  MeasurementFcn2=myMeasurementFcn  HasMeasurementEnablePort2=off  HasAdditiveMeasurementNoise2=Additive  MeasurementNoise2=1  HasTimeVaryingMeasurementNoise2=off  HasMeasurementFcnExtraArgument2=0  HasMeasurementWrapping2=off  MeasurementFcn3=myMeasurementFcn  HasMeasurementEnablePort3=off  HasAdditiveMeasurementNoise3=Additive  MeasurementNoise3=1  HasTimeVaryingMeasurementNoise3=off  HasMeasurementFcnExtraArgument3=0  HasMeasurementWrapping3=off  MeasurementFcn4=myMeasurementFcn  HasMeasurementEnablePort4=off  HasAdditiveMeasurementNoise4=Additive  MeasurementNoise4=1  HasTimeVaryingMeasurementNoise4=off  HasMeasurementFcnExtraArgument4=0  HasMeasurementWrapping4=off  MeasurementFcn5=myMeasurementFcn  HasMeasurementEnablePort5=off  HasAdditiveMeasurementNoise5=Additive  MeasurementNoise5=1  HasTimeVaryingMeasurementNoise5=off  HasMeasurementFcnExtraArgument5=0  HasMeasurementWrapping5=off  EnableMultirate=off  StateTransitionFcnSampleTime=-1  MeasurementFcn1SampleTime=-1  MeasurementFcn2SampleTime=-1  MeasurementFcn3SampleTime=-1  MeasurementFcn4SampleTime=-1  MeasurementFcn5SampleTime=-1  UseCurrentEstimator=on  OutputStateCovariance=off  DataType=single  SampleTime=ts_controller  NumberOfMeasurements=1
  SOC_UKF : Outport  VectorParamsAs1DForOutWhenUnconnected=off
  SOC_EKF : Outport  Port=2  VectorParamsAs1DForOutWhenUnconnected=off
  wires:
  UKF/1 -> SOC1/1
  Cell_Voltage/1 -> UKF/1, EKF/1
  SOC1/1 -> SOC_UKF/1  "SOC_UKF"
  EKF/1 -> SOC/1
  SOC/1 -> SOC_EKF/1  "SOC_EKF"

== system eVTOL_System/Battery System/Battery/HW Interface/BCE - HIL/Battery Cell Emulator/BCE Bus Packing  ==
  Cell 1 Enable : Inport
  Cell 2 Enable : Inport  Port=2
  Cell 3 Enable : Inport  Port=3
  Cell 4 Enable : Inport  Port=4
  Cell 5 Enable : Inport  Port=5
  Cell 6 Enable : Inport  Port=6
  Cell 7 Enable : Inport  Port=7
  Cell 8 Enable : Inport  Port=8
  Cell 9 Enable : Inport  Port=9
  Cell 10 Enable : Inport  Port=10
  Cell 11 Enable : Inport  Port=11
  Cell 12 Enable : Inport  Port=12
  Cell 12 Voltage : Inport  Port=13
  Cell 11 Voltage : Inport  Port=14
  Cell 10 Voltage : Inport  Port=15
  Cell 9 Voltage : Inport  Port=16
  Cell 8 Voltage : Inport  Port=17
  Cell 7 Voltage : Inport  Port=18
  Cell 6 Voltage : Inport  Port=19
  Cell 5 Voltage : Inport  Port=20
  Cell 4 Voltage : Inport  Port=21
  Cell 3 Voltage : Inport  Port=22
  Cell 2 Voltage : Inport  Port=23
  Cell 1 Voltage : Inport  Port=24
  Cell 1 Current : Inport  Port=25
  Cell 2 Current : Inport  Port=26
  Cell 3 Current : Inport  Port=27
  Cell 4 Current : Inport  Port=28
  Cell 5 Current : Inport  Port=29
  Cell 6 Current : Inport  Port=30
  Cell 7 Current : Inport  Port=31
  Cell 8 Current : Inport  Port=32
  Cell 9 Current : Inport  Port=33
  Cell 10 Current : Inport  Port=34
  Cell 11 Current : Inport  Port=35
  Cell 12 Current : Inport  Port=36
  Bus Assignment : BusAssignment  AssignedSignals=Cell_1.Enable,Cell_2.Enable,Cell_3.Enable,Cell_4.Enable,Cell_5.Enable,Cell_6.Enable,Cell_7.Enable,Cell_8.Enable,Cell_9.Enable,Cell_10.Enable,Cell_11.Enable,Cell_12.Enable,Cell_1.V,Cell_2.V,Cell_3.V,Cell_4.V,Cell_5.V,Cell_6.V,Cell_7.V,Cell_8.V,Cell_9.V,Cell_10.V,Cell_11.V,Cell_12.V,Cell_1.I,Cell_2.I,Cell_3.I,Cell_4.I,Cell_5.I,Cell_6.I,Cell_7.I,Cell_8.I,Cell_9.I,Cell_10.I,Cell_11.I,Cell_12.I
  Constant : Constant  Value=BCE_Set_init  OutDataTypeStr=Bus: BCE_Set
  BCE Bus : Outport
  wires:
  Cell 11 Enable/1 -> Bus Assignment/12
  Cell 11 Voltage/1 -> Bus Assignment/24
  Cell 11 Current/1 -> Bus Assignment/36
  Cell 12 Current/1 -> Bus Assignment/37
  Cell 12 Voltage/1 -> Bus Assignment/25
  Cell 12 Enable/1 -> Bus Assignment/13
  Cell 10 Enable/1 -> Bus Assignment/11
  Cell 10 Voltage/1 -> Bus Assignment/23
  Cell 10 Current/1 -> Bus Assignment/35
  Cell 9 Current/1 -> Bus Assignment/34
  Cell 9 Voltage/1 -> Bus Assignment/22
  Cell 9 Enable/1 -> Bus Assignment/10
  Cell 5 Enable/1 -> Bus Assignment/6
  Cell 5 Voltage/1 -> Bus Assignment/18
  Cell 5 Current/1 -> Bus Assignment/30
  Cell 6 Current/1 -> Bus Assignment/31
  Cell 6 Voltage/1 -> Bus Assignment/19
  Cell 6 Enable/1 -> Bus Assignment/7
  Cell 8 Enable/1 -> Bus Assignment/9
  Cell 8 Voltage/1 -> Bus Assignment/21
  Cell 8 Current/1 -> Bus Assignment/33
  Cell 7 Current/1 -> Bus Assignment/32
  Cell 7 Voltage/1 -> Bus Assignment/20
  Cell 7 Enable/1 -> Bus Assignment/8
  Cell 3 Enable/1 -> Bus Assignment/4
  Cell 3 Voltage/1 -> Bus Assignment/16
  Cell 3 Current/1 -> Bus Assignment/28
  Cell 4 Current/1 -> Bus Assignment/29
  Cell 4 Voltage/1 -> Bus Assignment/17
  Cell 4 Enable/1 -> Bus Assignment/5
  Cell 2 Enable/1 -> Bus Assignment/3
  Cell 2 Voltage/1 -> Bus Assignment/15
  Cell 2 Current/1 -> Bus Assignment/27
  Cell 1 Current/1 -> Bus Assignment/26
  Cell 1 Enable/1 -> Bus Assignment/2
  Bus Assignment/1 -> BCE Bus/1
  Constant/1 -> Bus Assignment/1
  Cell 1 Voltage/1 -> Bus Assignment/14

== system eVTOL_System/Battery System/Battery/HW Interface/BCE - HIL/Battery Cell Emulator/BCE Bus Packing 1 ==
  Cell 1 Enable : Inport
  Cell 2 Enable : Inport  Port=2
  Cell 3 Enable : Inport  Port=3
  Cell 4 Enable : Inport  Port=4
  Cell 5 Enable : Inport  Port=5
  Cell 6 Enable : Inport  Port=6
  Cell 7 Enable : Inport  Port=7
  Cell 8 Enable : Inport  Port=8
  Cell 9 Enable : Inport  Port=9
  Cell 10 Enable : Inport  Port=10
  Cell 11 Enable : Inport  Port=11
  Cell 12 Enable : Inport  Port=12
  Cell 12 Voltage : Inport  Port=13
  Cell 11 Voltage : Inport  Port=14
  Cell 10 Voltage : Inport  Port=15
  Cell 9 Voltage : Inport  Port=16
  Cell 8 Voltage : Inport  Port=17
  Cell 7 Voltage : Inport  Port=18
  Cell 6 Voltage : Inport  Port=19
  Cell 5 Voltage : Inport  Port=20
  Cell 4 Voltage : Inport  Port=21
  Cell 3 Voltage : Inport  Port=22
  Cell 2 Voltage : Inport  Port=23
  Cell 1 Voltage : Inport  Port=24
  Cell 1 Current : Inport  Port=25
  Cell 2 Current : Inport  Port=26
  Cell 3 Current : Inport  Port=27
  Cell 4 Current : Inport  Port=28
  Cell 5 Current : Inport  Port=29
  Cell 6 Current : Inport  Port=30
  Cell 7 Current : Inport  Port=31
  Cell 8 Current : Inport  Port=32
  Cell 9 Current : Inport  Port=33
  Cell 10 Current : Inport  Port=34
  Cell 11 Current : Inport  Port=35
  Cell 12 Current : Inport  Port=36
  Bus Assignment : BusAssignment  AssignedSignals=Cell_1.Enable,Cell_2.Enable,Cell_3.Enable,Cell_4.Enable,Cell_5.Enable,Cell_6.Enable,Cell_7.Enable,Cell_8.Enable,Cell_9.Enable,Cell_10.Enable,Cell_11.Enable,Cell_12.Enable,Cell_1.V,Cell_2.V,Cell_3.V,Cell_4.V,Cell_5.V,Cell_6.V,Cell_7.V,Cell_8.V,Cell_9.V,Cell_10.V,Cell_11.V,Cell_12.V,Cell_1.I,Cell_2.I,Cell_3.I,Cell_4.I,Cell_5.I,Cell_6.I,Cell_7.I,Cell_8.I,Cell_9.I,Cell_10.I,Cell_11.I,Cell_12.I
  Constant : Constant  Value=BCE_Set_init  OutDataTypeStr=Bus: BCE_Set
  BCE Bus : Outport
  wires:
  Cell 11 Enable/1 -> Bus Assignment/12
  Cell 11 Voltage/1 -> Bus Assignment/24
  Cell 11 Current/1 -> Bus Assignment/36
  Cell 12 Current/1 -> Bus Assignment/37
  Cell 12 Voltage/1 -> Bus Assignment/25
  Cell 12 Enable/1 -> Bus Assignment/13
  Cell 10 Enable/1 -> Bus Assignment/11
  Cell 10 Voltage/1 -> Bus Assignment/23
  Cell 10 Current/1 -> Bus Assignment/35
  Cell 9 Current/1 -> Bus Assignment/34
  Cell 9 Voltage/1 -> Bus Assignment/22
  Cell 9 Enable/1 -> Bus Assignment/10
  Cell 5 Enable/1 -> Bus Assignment/6
  Cell 5 Voltage/1 -> Bus Assignment/18
  Cell 5 Current/1 -> Bus Assignment/30
  Cell 6 Current/1 -> Bus Assignment/31
  Cell 6 Voltage/1 -> Bus Assignment/19
  Cell 6 Enable/1 -> Bus Assignment/7
  Cell 8 Enable/1 -> Bus Assignment/9
  Cell 8 Voltage/1 -> Bus Assignment/21
  Cell 8 Current/1 -> Bus Assignment/33
  Cell 7 Current/1 -> Bus Assignment/32
  Cell 7 Voltage/1 -> Bus Assignment/20
  Cell 7 Enable/1 -> Bus Assignment/8
  Cell 3 Enable/1 -> Bus Assignment/4
  Cell 3 Voltage/1 -> Bus Assignment/16
  Cell 3 Current/1 -> Bus Assignment/28
  Cell 4 Current/1 -> Bus Assignment/29
  Cell 4 Voltage/1 -> Bus Assignment/17
  Cell 4 Enable/1 -> Bus Assignment/5
  Cell 2 Enable/1 -> Bus Assignment/3
  Cell 2 Voltage/1 -> Bus Assignment/15
  Cell 2 Current/1 -> Bus Assignment/27
  Cell 1 Current/1 -> Bus Assignment/26
  Cell 1 Enable/1 -> Bus Assignment/2
  Bus Assignment/1 -> BCE Bus/1
  Constant/1 -> Bus Assignment/1
  Cell 1 Voltage/1 -> Bus Assignment/14

== system eVTOL_System/Battery System/Battery/HW Interface/BCE - HIL/Battery Cell Emulator/BCE Read  ==
  Subsystem : Subsystem
  Data : Outport  OutDataTypeStr=Bus: BCE_Get
  wires:
  Subsystem/1(Data) -> Data/1

== system eVTOL_System/Battery System/Battery/HW Interface/BCE - HIL/Battery Cell Emulator/BCE Read 1 ==
  Subsystem : Subsystem
  Data : Outport  OutDataTypeStr=Bus: BCE_Get
  wires:
  Subsystem/1(Data) -> Data/1

== system eVTOL_System/Battery System/Battery/HW Interface/BCE - HIL/Battery Cell Emulator/BCE Setup  ==
  EtherCAT Init : slrealtimeethercatlib/EtherCAT Init  Priority=0  config_file=C:\Users\jatin.anand\AppData\Local\Temp\sg_bmts\VTOLTiltrotor\sg_bmts_ENI_bus0.xml  device_id=0  portnum=1  initstate=2  dctuning=0  enaDebug=0  logFile='c:\dbglog.txt'  sample_time=0.001000  DCMode=0
  Terminator : Terminator
  wires:
  EtherCAT Init/1 -> Terminator/1

== system eVTOL_System/Battery System/Battery/HW Interface/BCE - HIL/Battery Cell Emulator/BCE Write  ==
  Data : Inport  OutDataTypeStr=Bus: BCE_Set
  Subsystem : Subsystem
  wires:
  Data/1 -> Subsystem/1(Data)

== system eVTOL_System/Battery System/Battery/HW Interface/BCE - HIL/Battery Cell Emulator/BCE Write 1 ==
  Data : Inport  OutDataTypeStr=Bus: BCE_Set
  Subsystem : Subsystem
  wires:
  Data/1 -> Subsystem/1(Data)

== system eVTOL_System/Battery System/Battery/HW Interface/BCE - HIL/Battery Cell Emulator/Selector ==
  In1 : Inport
  Demux : Demux  Outputs=24
  Mux : Mux  Inputs=12
  Out1 : Outport
  wires:
  In1/1 -> Demux/1
  Mux/1 -> Out1/1
  Demux/1 -> Mux/1
  Demux/2 -> Mux/2
  Demux/3 -> Mux/3
  Demux/4 -> Mux/4
  Demux/5 -> Mux/5
  Demux/6 -> Mux/6
  Demux/7 -> Mux/7
  Demux/8 -> Mux/8
  Demux/9 -> Mux/9
  Demux/10 -> Mux/10
  Demux/11 -> Mux/11
  Demux/12 -> Mux/12

== system eVTOL_System/Battery System/Battery/HW Interface/BCE - HIL/Battery Cell Emulator/Selector1 ==
  In1 : Inport
  Demux : Demux  Outputs=24
  Mux : Mux  Inputs=12
  Out1 : Outport
  wires:
  In1/1 -> Demux/1
  Demux/13 -> Mux/1
  Demux/14 -> Mux/2
  Demux/15 -> Mux/3
  Demux/16 -> Mux/4
  Demux/17 -> Mux/5
  Demux/18 -> Mux/6
  Demux/19 -> Mux/7
  Demux/20 -> Mux/8
  Demux/21 -> Mux/9
  Demux/22 -> Mux/10
  Demux/23 -> Mux/11
  Demux/24 -> Mux/12
  Mux/1 -> Out1/1

== system eVTOL_System/Battery System/Battery/HW Interface/BCE - HIL/Battery Cell Emulator/Selector2 ==
  In1 : Inport
  Bus Selector1 : BusSelector  OutputSignals=Cell_Voltages
  Demux : Demux  Outputs=100
  Mux : Mux  Inputs=24
  Out1 : Outport
  wires:
  Bus Selector1/1 -> Demux/1  "<Cell_Voltages>"
  Mux/1 -> Out1/1
  In1/1 -> Bus Selector1/1
  Demux/1 -> Mux/1
  Demux/2 -> Mux/2
  Demux/3 -> Mux/3
  Demux/4 -> Mux/4
  Demux/5 -> Mux/5
  Demux/6 -> Mux/6
  Demux/7 -> Mux/7
  Demux/8 -> Mux/8
  Demux/9 -> Mux/9
  Demux/10 -> Mux/10
  Demux/11 -> Mux/11
  Demux/12 -> Mux/12
  Demux/13 -> Mux/13
  Demux/14 -> Mux/14
  Demux/15 -> Mux/15
  Demux/16 -> Mux/16
  Demux/17 -> Mux/17
  Demux/18 -> Mux/18
  Demux/19 -> Mux/19
  Demux/20 -> Mux/20
  Demux/21 -> Mux/21
  Demux/22 -> Mux/22
  Demux/23 -> Mux/23
  Demux/24 -> Mux/24

== system eVTOL_System/Battery System/Battery/HW Interface/BCE - HIL/Battery Cell Emulator/Selector3 ==
  In1 : Inport
  Bus Selector1 : BusSelector  OutputSignals=Cell_Voltages
  Demux : Demux  Outputs=100
  Mux : Mux  Inputs=24
  Mux1 : Mux  Inputs=76
  Terminator : Terminator
  Out1 : Outport
  wires:
  Bus Selector1/1 -> Demux/1  "<Cell_Voltages>"
  In1/1 -> Bus Selector1/1
  Demux/1 -> Mux/1
  Demux/2 -> Mux/2
  Demux/3 -> Mux/3
  Demux/4 -> Mux/4
  Demux/5 -> Mux/5
  Demux/6 -> Mux/6
  Demux/7 -> Mux/7
  Demux/8 -> Mux/8
  Demux/9 -> Mux/9
  Demux/10 -> Mux/10
  Demux/11 -> Mux/11
  Demux/12 -> Mux/12
  Demux/13 -> Mux/13
  Demux/14 -> Mux/14
  Demux/15 -> Mux/15
  Demux/16 -> Mux/16
  Demux/17 -> Mux/17
  Demux/18 -> Mux/18
  Demux/19 -> Mux/19
  Demux/20 -> Mux/20
  Demux/21 -> Mux/21
  Demux/22 -> Mux/22
  Demux/23 -> Mux/23
  Demux/24 -> Mux/24
  Demux/25 -> Mux1/1
  Demux/26 -> Mux1/2
  Demux/27 -> Mux1/3
  Demux/28 -> Mux1/4
  Demux/29 -> Mux1/5
  Demux/30 -> Mux1/6
  Demux/31 -> Mux1/7
  Demux/32 -> Mux1/8
  Demux/33 -> Mux1/9
  Demux/34 -> Mux1/10
  Demux/35 -> Mux1/11
  Demux/36 -> Mux1/12
  Demux/37 -> Mux1/13
  Demux/38 -> Mux1/14
  Demux/39 -> Mux1/15
  Demux/40 -> Mux1/16
  Demux/41 -> Mux1/17
  Demux/42 -> Mux1/18
  Demux/43 -> Mux1/19
  Demux/44 -> Mux1/20
  Demux/45 -> Mux1/21
  Demux/46 -> Mux1/22
  Demux/47 -> Mux1/23
  Demux/48 -> Mux1/24
  Demux/49 -> Mux1/25
  Demux/50 -> Mux1/26
  Demux/51 -> Mux1/27
  Demux/52 -> Mux1/28
  Demux/53 -> Mux1/29
  Demux/54 -> Mux1/30
  Demux/55 -> Mux1/31
  Demux/56 -> Mux1/32
  Demux/57 -> Mux1/33
  Demux/58 -> Mux1/34
  Demux/59 -> Mux1/35
  Demux/60 -> Mux1/36
  Demux/61 -> Mux1/37
  Demux/62 -> Mux1/38
  Demux/63 -> Mux1/39
  Demux/64 -> Mux1/40
  Demux/65 -> Mux1/41
  Demux/66 -> Mux1/42
  Demux/67 -> Mux1/43
  Demux/68 -> Mux1/44
  Demux/69 -> Mux1/45
  Demux/70 -> Mux1/46
  Demux/71 -> Mux1/47
  Demux/72 -> Mux1/48
  Demux/73 -> Mux1/49
  Demux/74 -> Mux1/50
  Demux/75 -> Mux1/51
  Demux/76 -> Mux1/52
  Demux/77 -> Mux1/53
  Demux/78 -> Mux1/54
  Demux/79 -> Mux1/55
  Demux/80 -> Mux1/56
  Demux/81 -> Mux1/57
  Demux/82 -> Mux1/58
  Demux/83 -> Mux1/59
  Demux/84 -> Mux1/60
  Demux/85 -> Mux1/61
  Demux/86 -> Mux1/62
  Demux/87 -> Mux1/63
  Demux/88 -> Mux1/64
  Demux/89 -> Mux1/65
  Demux/90 -> Mux1/66
  Demux/91 -> Mux1/67
  Demux/92 -> Mux1/68
  Demux/93 -> Mux1/69
  Demux/94 -> Mux1/70
  Demux/95 -> Mux1/71
  Demux/96 -> Mux1/72
  Demux/97 -> Mux1/73
  Demux/98 -> Mux1/74
  Demux/99 -> Mux1/75
  Demux/100 -> Mux1/76
  Mux1/1 -> Out1/1
  Mux/1 -> Terminator/1

== system eVTOL_System/Dynamics/Force and Moments/Aerodynamic Forces/Compute Body Frame Forces and Moments/Rotate FM to body frame/Rotate Forces ==
  F_w : Inport
  alpha_beta : Inport  Port=2
  Product2 : Product  Multiplication=Matrix(*)  SaturateOnIntegerOverflow=on  OutDataTypeStr=Inherit: Same as first input
  RB2W : Subsystem
  RW2B : Math  Operator=transpose  SignedPower=on
  F_b : Outport  PortDimensions=3  VectorParamsAs1DForOutWhenUnconnected=off
  wires:
  RW2B/1 -> Product2/1
  F_w/1 -> Product2/2
  Product2/1 -> F_b/1
  alpha_beta/1 -> RB2W/1(aoa beta)
  RB2W/1(Rw2b) -> RW2B/1

== system eVTOL_System/Dynamics/Force and Moments/Aerodynamic Forces/Compute Body Frame Forces and Moments/Rotate FM to body frame/Rotate Moments ==
  alpha_beta : Inport
  M_w : Inport  Port=2
  Product2 : Product  Multiplication=Matrix(*)  SaturateOnIntegerOverflow=on  OutDataTypeStr=Inherit: Same as first input
  RB2W : Subsystem
  RW2B : Math  Operator=transpose  SignedPower=on
  M_b : Outport  PortDimensions=3  VectorParamsAs1DForOutWhenUnconnected=off
  wires:
  RW2B/1 -> Product2/1
  RB2W/1(Rw2b) -> RW2B/1
  alpha_beta/1 -> RB2W/1(aoa beta)
  Product2/1 -> M_b/1
  M_w/1 -> Product2/2
